simulink model "Second_AGC"  (R2022a)
settings: Solver=FixedStepDiscrete  StartTime=0.0  StopTime=Time*20000  RelTol=1e-3
PreLoadFcn:
  | clc,clear,close all
  | 
  | F               = 1e1;
  | Fs              = 200e6;
  | Frame           = 1  ;
  | Amplitudes      = [0.1,1,0.5,1,0.25];
  | R               = 2;
  | a               = 0.01;
  | alpha           = 0.4;
  | NumFrames       = length(Amplitudes);
  | SamplesY        = [];
  | TimeAxis        = [];
  | NumSym          = 1e3;
  | NumBitsInSymbol = 4;
  | sps             = 4;
  | rolloff         = 0.3;
  | span            = 32;
  | 
  | SQRRC = rcosdesign(rolloff, span, sps);
  | delay = mean(grpdelay(SQRRC));
  | for i = 1:NumFrames
  |     x = randi([0 3],NumSym,1);
  |     QPSK   = qammod(x,NumBitsInSymbol);
  |     Signal = Amplitudes(i) * upfirdn(QPSK, SQRRC, sps);
  |      Signal(1:delay-1)     = [];
  |      Signal(end-delay+3:end) = [];
  |     SamplesY = [SamplesY; Signal];
  | end
  | SamplesY = SamplesY.';
  | FixedRe = fi(real(SamplesY),1,16,14);
  | FixedIm = fi(imag(SamplesY),1,16,14);
  | FixedR  = fi(R,0,2,0);
  | Fixeda  = fi(a,1,13,12);
  | RealSimpleAGC = real(SamplesY);
  | ImagSimpleAGC = imag(SamplesY);
InitFcn:
  | Time = 40;
  | PowerDelay = Time*100;
libraries: sim_stud_lib_r2022a x25, dspsrcs4 x14, dspsigops x10, dspswit3 x5
(part 2 of 2)

== system Second_AGC/Calculation of average power1/MA and divide input /fpga_dfe3 ==
  ena : Inport
  d : Inport  Port=2
  Delay16 : Delay  DelayLength=1
  Enabled Subsystem : Subsystem  TreatAsAtomicUnit=on
  q : Outport  VectorParamsAs1DForOutWhenUnconnected=off
  wires:
  Enabled Subsystem/1(Out1) -> Delay16/1
  Delay16/1 -> q/1
  ena/1 -> Enabled Subsystem/Enable
  d/1 -> Enabled Subsystem/1(In1)

== system Second_AGC/Compare different clk//input/FPGA-orieded Lyons/Clock 1 ==
  ena : Inport
  d : Inport  Port=2
  Delay16 : Delay  DelayLength=1
  Enabled Subsystem : sim_stud_lib_r2022a/fpga_dfe/Enabled Subsystem  SystemSampleTime=-1  VariantActivationTime=update diagram  Latency=0  AutoFrameSizeCalculation=off
  q : Outport  VectorParamsAs1DForOutWhenUnconnected=off
  wires:
  Delay16/1 -> q/1
  d/1 -> Enabled Subsystem/1
  Enabled Subsystem/1 -> Delay16/1
  ena/1 -> Enabled Subsystem/Enable

== system Second_AGC/Compare different clk//input/FPGA-orieded Lyons/Clock 2 ==
  ena : Inport
  d : Inport  Port=2
  Delay16 : Delay  DelayLength=1
  Enabled Subsystem : sim_stud_lib_r2022a/fpga_dfe/Enabled Subsystem  SystemSampleTime=-1  VariantActivationTime=update diagram  Latency=0  AutoFrameSizeCalculation=off
  q : Outport  VectorParamsAs1DForOutWhenUnconnected=off
  wires:
  Delay16/1 -> q/1
  d/1 -> Enabled Subsystem/1
  Enabled Subsystem/1 -> Delay16/1
  ena/1 -> Enabled Subsystem/Enable

== system Second_AGC/Compare different clk//input/FPGA-orieded Lyons/Clock 3 ==
  ena : Inport
  d : Inport  Port=2
  Delay16 : Delay  DelayLength=1
  Enabled Subsystem : sim_stud_lib_r2022a/fpga_dfe/Enabled Subsystem  SystemSampleTime=-1  VariantActivationTime=update diagram  Latency=0  AutoFrameSizeCalculation=off
  q : Outport  VectorParamsAs1DForOutWhenUnconnected=off
  wires:
  Delay16/1 -> q/1
  d/1 -> Enabled Subsystem/1
  Enabled Subsystem/1 -> Delay16/1
  ena/1 -> Enabled Subsystem/Enable

== system Second_AGC/Compare different clk//input/FPGA-orieded Lyons/Clock 4 ==
  ena : Inport
  d : Inport  Port=2
  Delay16 : Delay  DelayLength=1
  Enabled Subsystem : sim_stud_lib_r2022a/fpga_dfe/Enabled Subsystem  SystemSampleTime=-1  VariantActivationTime=update diagram  Latency=0  AutoFrameSizeCalculation=off
  q : Outport  VectorParamsAs1DForOutWhenUnconnected=off
  wires:
  Delay16/1 -> q/1
  d/1 -> Enabled Subsystem/1
  Enabled Subsystem/1 -> Delay16/1
  ena/1 -> Enabled Subsystem/Enable

== system Second_AGC/Compare different clk//input/FPGA-orieded Lyons/Clock 5 ==
  ena : Inport
  d : Inport  Port=2
  Delay16 : Delay  DelayLength=1
  Enabled Subsystem : sim_stud_lib_r2022a/fpga_dfe/Enabled Subsystem  SystemSampleTime=-1  VariantActivationTime=update diagram  Latency=0  AutoFrameSizeCalculation=off
  q : Outport  VectorParamsAs1DForOutWhenUnconnected=off
  wires:
  Delay16/1 -> q/1
  d/1 -> Enabled Subsystem/1
  Enabled Subsystem/1 -> Delay16/1
  ena/1 -> Enabled Subsystem/Enable

== system Second_AGC/Compare different clk//input/FPGA-orieded Lyons/fpga_dfe ==
  ena : Inport
  d : Inport  Port=2
  Delay16 : Delay  DelayLength=1
  Enabled Subsystem : Subsystem  TreatAsAtomicUnit=on
  q : Outport  VectorParamsAs1DForOutWhenUnconnected=off
  wires:
  Enabled Subsystem/1(Out1) -> Delay16/1
  Delay16/1 -> q/1
  ena/1 -> Enabled Subsystem/Enable
  d/1 -> Enabled Subsystem/1(In1)

== system Second_AGC/Compare different clk//input/FPGA-orieded Lyons/fpga_dfe1 ==
  ena : Inport
  d : Inport  Port=2
  Delay16 : Delay  DelayLength=1
  Enabled Subsystem : Subsystem  TreatAsAtomicUnit=on
  q : Outport  VectorParamsAs1DForOutWhenUnconnected=off
  wires:
  Enabled Subsystem/1(Out1) -> Delay16/1
  Delay16/1 -> q/1
  ena/1 -> Enabled Subsystem/Enable
  d/1 -> Enabled Subsystem/1(In1)

== system Second_AGC/Compare different clk//input/FPGA-orieded Lyons/fpga_dfe2 ==
  ena : Inport
  d : Inport  Port=2
  Delay16 : Delay  DelayLength=1
  Enabled Subsystem : Subsystem  TreatAsAtomicUnit=on
  q : Outport  VectorParamsAs1DForOutWhenUnconnected=off
  wires:
  Enabled Subsystem/1(Out1) -> Delay16/1
  Delay16/1 -> q/1
  ena/1 -> Enabled Subsystem/Enable
  d/1 -> Enabled Subsystem/1(In1)

== system Second_AGC/Compare different clk//input/FPGA-orieded Lyons/fpga_dfe3 ==
  ena : Inport
  d : Inport  Port=2
  Delay16 : Delay  DelayLength=1
  Enabled Subsystem : Subsystem  TreatAsAtomicUnit=on
  q : Outport  VectorParamsAs1DForOutWhenUnconnected=off
  wires:
  Enabled Subsystem/1(Out1) -> Delay16/1
  Delay16/1 -> q/1
  ena/1 -> Enabled Subsystem/Enable
  d/1 -> Enabled Subsystem/1(In1)

== system Second_AGC/Compare different clk//input/FPGA-orieded Lyons1/Clock 1 ==
  ena : Inport
  d : Inport  Port=2
  Delay16 : Delay  DelayLength=1
  Enabled Subsystem : sim_stud_lib_r2022a/fpga_dfe/Enabled Subsystem  SystemSampleTime=-1  VariantActivationTime=update diagram  Latency=0  AutoFrameSizeCalculation=off
  q : Outport  VectorParamsAs1DForOutWhenUnconnected=off
  wires:
  Delay16/1 -> q/1
  d/1 -> Enabled Subsystem/1
  Enabled Subsystem/1 -> Delay16/1
  ena/1 -> Enabled Subsystem/Enable

== system Second_AGC/Compare different clk//input/FPGA-orieded Lyons1/Clock 2 ==
  ena : Inport
  d : Inport  Port=2
  Delay16 : Delay  DelayLength=1
  Enabled Subsystem : sim_stud_lib_r2022a/fpga_dfe/Enabled Subsystem  SystemSampleTime=-1  VariantActivationTime=update diagram  Latency=0  AutoFrameSizeCalculation=off
  q : Outport  VectorParamsAs1DForOutWhenUnconnected=off
  wires:
  Delay16/1 -> q/1
  d/1 -> Enabled Subsystem/1
  Enabled Subsystem/1 -> Delay16/1
  ena/1 -> Enabled Subsystem/Enable

== system Second_AGC/Compare different clk//input/FPGA-orieded Lyons1/Clock 3 ==
  ena : Inport
  d : Inport  Port=2
  Delay16 : Delay  DelayLength=1
  Enabled Subsystem : sim_stud_lib_r2022a/fpga_dfe/Enabled Subsystem  SystemSampleTime=-1  VariantActivationTime=update diagram  Latency=0  AutoFrameSizeCalculation=off
  q : Outport  VectorParamsAs1DForOutWhenUnconnected=off
  wires:
  Delay16/1 -> q/1
  d/1 -> Enabled Subsystem/1
  Enabled Subsystem/1 -> Delay16/1
  ena/1 -> Enabled Subsystem/Enable

== system Second_AGC/Compare different clk//input/FPGA-orieded Lyons1/Clock 4 ==
  ena : Inport
  d : Inport  Port=2
  Delay16 : Delay  DelayLength=1
  Enabled Subsystem : sim_stud_lib_r2022a/fpga_dfe/Enabled Subsystem  SystemSampleTime=-1  VariantActivationTime=update diagram  Latency=0  AutoFrameSizeCalculation=off
  q : Outport  VectorParamsAs1DForOutWhenUnconnected=off
  wires:
  Delay16/1 -> q/1
  d/1 -> Enabled Subsystem/1
  Enabled Subsystem/1 -> Delay16/1
  ena/1 -> Enabled Subsystem/Enable

== system Second_AGC/Compare different clk//input/FPGA-orieded Lyons1/Clock 5 ==
  ena : Inport
  d : Inport  Port=2
  Delay16 : Delay  DelayLength=1
  Enabled Subsystem : sim_stud_lib_r2022a/fpga_dfe/Enabled Subsystem  SystemSampleTime=-1  VariantActivationTime=update diagram  Latency=0  AutoFrameSizeCalculation=off
  q : Outport  VectorParamsAs1DForOutWhenUnconnected=off
  wires:
  Delay16/1 -> q/1
  d/1 -> Enabled Subsystem/1
  Enabled Subsystem/1 -> Delay16/1
  ena/1 -> Enabled Subsystem/Enable

== system Second_AGC/Compare different clk//input/FPGA-orieded Lyons1/fpga_dfe ==
  ena : Inport
  d : Inport  Port=2
  Delay16 : Delay  DelayLength=1
  Enabled Subsystem : Subsystem  TreatAsAtomicUnit=on
  q : Outport  VectorParamsAs1DForOutWhenUnconnected=off
  wires:
  Enabled Subsystem/1(Out1) -> Delay16/1
  Delay16/1 -> q/1
  ena/1 -> Enabled Subsystem/Enable
  d/1 -> Enabled Subsystem/1(In1)

== system Second_AGC/Compare different clk//input/FPGA-orieded Lyons1/fpga_dfe1 ==
  ena : Inport
  d : Inport  Port=2
  Delay16 : Delay  DelayLength=1
  Enabled Subsystem : Subsystem  TreatAsAtomicUnit=on
  q : Outport  VectorParamsAs1DForOutWhenUnconnected=off
  wires:
  Enabled Subsystem/1(Out1) -> Delay16/1
  Delay16/1 -> q/1
  ena/1 -> Enabled Subsystem/Enable
  d/1 -> Enabled Subsystem/1(In1)

== system Second_AGC/Compare different clk//input/FPGA-orieded Lyons1/fpga_dfe2 ==
  ena : Inport
  d : Inport  Port=2
  Delay16 : Delay  DelayLength=1
  Enabled Subsystem : Subsystem  TreatAsAtomicUnit=on
  q : Outport  VectorParamsAs1DForOutWhenUnconnected=off
  wires:
  Enabled Subsystem/1(Out1) -> Delay16/1
  Delay16/1 -> q/1
  ena/1 -> Enabled Subsystem/Enable
  d/1 -> Enabled Subsystem/1(In1)

== system Second_AGC/Compare different clk//input/FPGA-orieded Lyons1/fpga_dfe3 ==
  ena : Inport
  d : Inport  Port=2
  Delay16 : Delay  DelayLength=1
  Enabled Subsystem : Subsystem  TreatAsAtomicUnit=on
  q : Outport  VectorParamsAs1DForOutWhenUnconnected=off
  wires:
  Enabled Subsystem/1(Out1) -> Delay16/1
  Delay16/1 -> q/1
  ena/1 -> Enabled Subsystem/Enable
  d/1 -> Enabled Subsystem/1(In1)

== system Second_AGC/Compare different clk//input/FPGA-orieded Lyons2/Clock 1 ==
  ena : Inport
  d : Inport  Port=2
  Delay16 : Delay  DelayLength=1
  Enabled Subsystem : sim_stud_lib_r2022a/fpga_dfe/Enabled Subsystem  SystemSampleTime=-1  VariantActivationTime=update diagram  Latency=0  AutoFrameSizeCalculation=off
  q : Outport  VectorParamsAs1DForOutWhenUnconnected=off
  wires:
  Delay16/1 -> q/1
  d/1 -> Enabled Subsystem/1
  Enabled Subsystem/1 -> Delay16/1
  ena/1 -> Enabled Subsystem/Enable

== system Second_AGC/Compare different clk//input/FPGA-orieded Lyons2/Clock 2 ==
  ena : Inport
  d : Inport  Port=2
  Delay16 : Delay  DelayLength=1
  Enabled Subsystem : sim_stud_lib_r2022a/fpga_dfe/Enabled Subsystem  SystemSampleTime=-1  VariantActivationTime=update diagram  Latency=0  AutoFrameSizeCalculation=off
  q : Outport  VectorParamsAs1DForOutWhenUnconnected=off
  wires:
  Delay16/1 -> q/1
  d/1 -> Enabled Subsystem/1
  Enabled Subsystem/1 -> Delay16/1
  ena/1 -> Enabled Subsystem/Enable

== system Second_AGC/Compare different clk//input/FPGA-orieded Lyons2/Clock 3 ==
  ena : Inport
  d : Inport  Port=2
  Delay16 : Delay  DelayLength=1
  Enabled Subsystem : sim_stud_lib_r2022a/fpga_dfe/Enabled Subsystem  SystemSampleTime=-1  VariantActivationTime=update diagram  Latency=0  AutoFrameSizeCalculation=off
  q : Outport  VectorParamsAs1DForOutWhenUnconnected=off
  wires:
  Delay16/1 -> q/1
  d/1 -> Enabled Subsystem/1
  Enabled Subsystem/1 -> Delay16/1
  ena/1 -> Enabled Subsystem/Enable

== system Second_AGC/Compare different clk//input/FPGA-orieded Lyons2/Clock 4 ==
  ena : Inport
  d : Inport  Port=2
  Delay16 : Delay  DelayLength=1
  Enabled Subsystem : sim_stud_lib_r2022a/fpga_dfe/Enabled Subsystem  SystemSampleTime=-1  VariantActivationTime=update diagram  Latency=0  AutoFrameSizeCalculation=off
  q : Outport  VectorParamsAs1DForOutWhenUnconnected=off
  wires:
  Delay16/1 -> q/1
  d/1 -> Enabled Subsystem/1
  Enabled Subsystem/1 -> Delay16/1
  ena/1 -> Enabled Subsystem/Enable

== system Second_AGC/Compare different clk//input/FPGA-orieded Lyons2/Clock 5 ==
  ena : Inport
  d : Inport  Port=2
  Delay16 : Delay  DelayLength=1
  Enabled Subsystem : sim_stud_lib_r2022a/fpga_dfe/Enabled Subsystem  SystemSampleTime=-1  VariantActivationTime=update diagram  Latency=0  AutoFrameSizeCalculation=off
  q : Outport  VectorParamsAs1DForOutWhenUnconnected=off
  wires:
  Delay16/1 -> q/1
  d/1 -> Enabled Subsystem/1
  Enabled Subsystem/1 -> Delay16/1
  ena/1 -> Enabled Subsystem/Enable

== system Second_AGC/Compare different clk//input/FPGA-orieded Lyons2/fpga_dfe ==
  ena : Inport
  d : Inport  Port=2
  Delay16 : Delay  DelayLength=1
  Enabled Subsystem : Subsystem  TreatAsAtomicUnit=on
  q : Outport  VectorParamsAs1DForOutWhenUnconnected=off
  wires:
  Enabled Subsystem/1(Out1) -> Delay16/1
  Delay16/1 -> q/1
  ena/1 -> Enabled Subsystem/Enable
  d/1 -> Enabled Subsystem/1(In1)

== system Second_AGC/Compare different clk//input/FPGA-orieded Lyons2/fpga_dfe1 ==
  ena : Inport
  d : Inport  Port=2
  Delay16 : Delay  DelayLength=1
  Enabled Subsystem : Subsystem  TreatAsAtomicUnit=on
  q : Outport  VectorParamsAs1DForOutWhenUnconnected=off
  wires:
  Enabled Subsystem/1(Out1) -> Delay16/1
  Delay16/1 -> q/1
  ena/1 -> Enabled Subsystem/Enable
  d/1 -> Enabled Subsystem/1(In1)

== system Second_AGC/Compare different clk//input/FPGA-orieded Lyons2/fpga_dfe2 ==
  ena : Inport
  d : Inport  Port=2
  Delay16 : Delay  DelayLength=1
  Enabled Subsystem : Subsystem  TreatAsAtomicUnit=on
  q : Outport  VectorParamsAs1DForOutWhenUnconnected=off
  wires:
  Enabled Subsystem/1(Out1) -> Delay16/1
  Delay16/1 -> q/1
  ena/1 -> Enabled Subsystem/Enable
  d/1 -> Enabled Subsystem/1(In1)

== system Second_AGC/Compare different clk//input/FPGA-orieded Lyons2/fpga_dfe3 ==
  ena : Inport
  d : Inport  Port=2
  Delay16 : Delay  DelayLength=1
  Enabled Subsystem : Subsystem  TreatAsAtomicUnit=on
  q : Outport  VectorParamsAs1DForOutWhenUnconnected=off
  wires:
  Enabled Subsystem/1(Out1) -> Delay16/1
  Delay16/1 -> q/1
  ena/1 -> Enabled Subsystem/Enable
  d/1 -> Enabled Subsystem/1(In1)

== system Second_AGC/FPGA-orieded Lyons/fpga_dfe/Enabled Subsystem ==
  In1 : Inport
  Enable : EnablePort
  Out1 : Outport  VectorParamsAs1DForOutWhenUnconnected=off
  wires:
  In1/1 -> Out1/1

== system Second_AGC/FPGA-orieded Lyons/fpga_dfe1/Enabled Subsystem ==
  In1 : Inport
  Enable : EnablePort
  Out1 : Outport  VectorParamsAs1DForOutWhenUnconnected=off
  wires:
  In1/1 -> Out1/1

== system Second_AGC/FPGA-orieded Lyons/fpga_dfe2/Enabled Subsystem ==
  In1 : Inport
  Enable : EnablePort
  Out1 : Outport  VectorParamsAs1DForOutWhenUnconnected=off
  wires:
  In1/1 -> Out1/1

== system Second_AGC/FPGA-orieded Lyons/fpga_dfe3/Enabled Subsystem ==
  In1 : Inport
  Enable : EnablePort
  Out1 : Outport  VectorParamsAs1DForOutWhenUnconnected=off
  wires:
  In1/1 -> Out1/1

== system Second_AGC/Fixed Point FPGA-oriended Lyons/fpga_dfe/Enabled Subsystem ==
  In1 : Inport
  Enable : EnablePort
  Out1 : Outport  VectorParamsAs1DForOutWhenUnconnected=off
  wires:
  In1/1 -> Out1/1

== system Second_AGC/Fixed Point FPGA-oriended Lyons/fpga_dfe1/Enabled Subsystem ==
  In1 : Inport
  Enable : EnablePort
  Out1 : Outport  VectorParamsAs1DForOutWhenUnconnected=off
  wires:
  In1/1 -> Out1/1

== system Second_AGC/Fixed Point FPGA-oriended Lyons/fpga_dfe2/Enabled Subsystem ==
  In1 : Inport
  Enable : EnablePort
  Out1 : Outport  VectorParamsAs1DForOutWhenUnconnected=off
  wires:
  In1/1 -> Out1/1

== system Second_AGC/Fixed Point FPGA-oriended Lyons/fpga_dfe3/Enabled Subsystem ==
  In1 : Inport
  Enable : EnablePort
  Out1 : Outport  VectorParamsAs1DForOutWhenUnconnected=off
  wires:
  In1/1 -> Out1/1

== system Second_AGC/Calculation of average power/MA and divide AGC/fpga_dfe2/Enabled Subsystem ==
  In1 : Inport
  Enable : EnablePort
  Out1 : Outport  VectorParamsAs1DForOutWhenUnconnected=off
  wires:
  In1/1 -> Out1/1

== system Second_AGC/Calculation of average power/MA and divide AGC/fpga_dfe3/Enabled Subsystem ==
  In1 : Inport
  Enable : EnablePort
  Out1 : Outport  VectorParamsAs1DForOutWhenUnconnected=off
  wires:
  In1/1 -> Out1/1

== system Second_AGC/Calculation of average power/MA and divide input /fpga_dfe2/Enabled Subsystem ==
  In1 : Inport
  Enable : EnablePort
  Out1 : Outport  VectorParamsAs1DForOutWhenUnconnected=off
  wires:
  In1/1 -> Out1/1

== system Second_AGC/Calculation of average power/MA and divide input /fpga_dfe3/Enabled Subsystem ==
  In1 : Inport
  Enable : EnablePort
  Out1 : Outport  VectorParamsAs1DForOutWhenUnconnected=off
  wires:
  In1/1 -> Out1/1

== system Second_AGC/Calculation of average power1/MA and divide AGC/fpga_dfe2/Enabled Subsystem ==
  In1 : Inport
  Enable : EnablePort
  Out1 : Outport  VectorParamsAs1DForOutWhenUnconnected=off
  wires:
  In1/1 -> Out1/1

== system Second_AGC/Calculation of average power1/MA and divide AGC/fpga_dfe3/Enabled Subsystem ==
  In1 : Inport
  Enable : EnablePort
  Out1 : Outport  VectorParamsAs1DForOutWhenUnconnected=off
  wires:
  In1/1 -> Out1/1

== system Second_AGC/Calculation of average power1/MA and divide input /fpga_dfe2/Enabled Subsystem ==
  In1 : Inport
  Enable : EnablePort
  Out1 : Outport  VectorParamsAs1DForOutWhenUnconnected=off
  wires:
  In1/1 -> Out1/1

== system Second_AGC/Calculation of average power1/MA and divide input /fpga_dfe3/Enabled Subsystem ==
  In1 : Inport
  Enable : EnablePort
  Out1 : Outport  VectorParamsAs1DForOutWhenUnconnected=off
  wires:
  In1/1 -> Out1/1

== system Second_AGC/Compare different clk//input/FPGA-orieded Lyons/fpga_dfe/Enabled Subsystem ==
  In1 : Inport
  Enable : EnablePort
  Out1 : Outport  VectorParamsAs1DForOutWhenUnconnected=off
  wires:
  In1/1 -> Out1/1

== system Second_AGC/Compare different clk//input/FPGA-orieded Lyons/fpga_dfe1/Enabled Subsystem ==
  In1 : Inport
  Enable : EnablePort
  Out1 : Outport  VectorParamsAs1DForOutWhenUnconnected=off
  wires:
  In1/1 -> Out1/1

== system Second_AGC/Compare different clk//input/FPGA-orieded Lyons/fpga_dfe2/Enabled Subsystem ==
  In1 : Inport
  Enable : EnablePort
  Out1 : Outport  VectorParamsAs1DForOutWhenUnconnected=off
  wires:
  In1/1 -> Out1/1

== system Second_AGC/Compare different clk//input/FPGA-orieded Lyons/fpga_dfe3/Enabled Subsystem ==
  In1 : Inport
  Enable : EnablePort
  Out1 : Outport  VectorParamsAs1DForOutWhenUnconnected=off
  wires:
  In1/1 -> Out1/1

== system Second_AGC/Compare different clk//input/FPGA-orieded Lyons1/fpga_dfe/Enabled Subsystem ==
  In1 : Inport
  Enable : EnablePort
  Out1 : Outport  VectorParamsAs1DForOutWhenUnconnected=off
  wires:
  In1/1 -> Out1/1

== system Second_AGC/Compare different clk//input/FPGA-orieded Lyons1/fpga_dfe1/Enabled Subsystem ==
  In1 : Inport
  Enable : EnablePort
  Out1 : Outport  VectorParamsAs1DForOutWhenUnconnected=off
  wires:
  In1/1 -> Out1/1

== system Second_AGC/Compare different clk//input/FPGA-orieded Lyons1/fpga_dfe2/Enabled Subsystem ==
  In1 : Inport
  Enable : EnablePort
  Out1 : Outport  VectorParamsAs1DForOutWhenUnconnected=off
  wires:
  In1/1 -> Out1/1

== system Second_AGC/Compare different clk//input/FPGA-orieded Lyons1/fpga_dfe3/Enabled Subsystem ==
  In1 : Inport
  Enable : EnablePort
  Out1 : Outport  VectorParamsAs1DForOutWhenUnconnected=off
  wires:
  In1/1 -> Out1/1

== system Second_AGC/Compare different clk//input/FPGA-orieded Lyons2/fpga_dfe/Enabled Subsystem ==
  In1 : Inport
  Enable : EnablePort
  Out1 : Outport  VectorParamsAs1DForOutWhenUnconnected=off
  wires:
  In1/1 -> Out1/1

== system Second_AGC/Compare different clk//input/FPGA-orieded Lyons2/fpga_dfe1/Enabled Subsystem ==
  In1 : Inport
  Enable : EnablePort
  Out1 : Outport  VectorParamsAs1DForOutWhenUnconnected=off
  wires:
  In1/1 -> Out1/1

== system Second_AGC/Compare different clk//input/FPGA-orieded Lyons2/fpga_dfe2/Enabled Subsystem ==
  In1 : Inport
  Enable : EnablePort
  Out1 : Outport  VectorParamsAs1DForOutWhenUnconnected=off
  wires:
  In1/1 -> Out1/1

== system Second_AGC/Compare different clk//input/FPGA-orieded Lyons2/fpga_dfe3/Enabled Subsystem ==
  In1 : Inport
  Enable : EnablePort
  Out1 : Outport  VectorParamsAs1DForOutWhenUnconnected=off
  wires:
  In1/1 -> Out1/1
